simulink model "circuitbreaker_2"  (Simulink 5.1)
settings: Solver=ode23t  StartTime=0.0  StopTime=50  MaxStep=.02  RelTol=1e-3
undefined symbols (not defined in the file or in its folder): A, gcbh, powericon, sigbuilder_block
libraries: powerlib x4, simulink_extras x1, powerlib_models x1
settings Model: LastModifiedBy=Owner  BooleanDataType=on  ProdHWDeviceType=Microprocessor

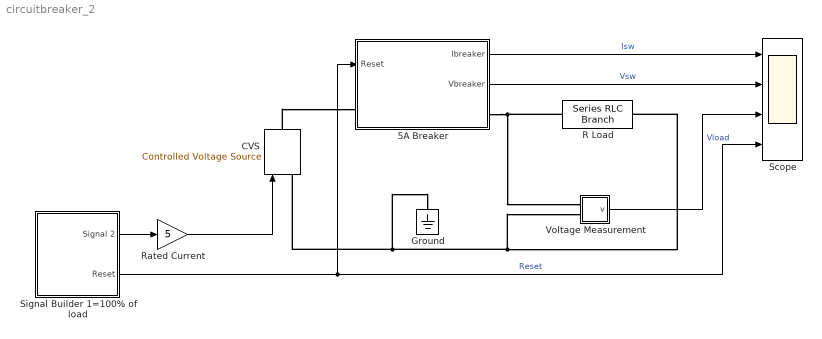
== system circuitbreaker_2 ==
  5A Breaker : Subsystem  mask{Iset=5, Tau=7}
      mask prompts: Iset "Current Rating (Amps)"; Tau "Mechanical Time Constant (Sec)"
  CVS : powerlib/Electrical Sources/Controlled Voltage Source  Description=source block  Orientation=up  Initialize=off  Amplitude=0  Phase=0  Frequency=60  Measurements=None
      settings: AttributesFormatString=\n
  Ground : powerlib/Elements/Ground  Orientation=down  PhysicalDomain=powersysdomain  SubClassName=unknown  PortType=p1  LConnTagsString=a
  R Load : powerlib/Elements/Series RLC Branch  PhysicalDomain=powersysdomain  SubClassName=unknown  PortType=p1  LConnTagsString=__new0  RConnTagsString=__new0  Resistance=1  Inductance=0  Capacitance=inf  Measurements=None
  Rated Current : Gain  Gain=5  SaturateOnIntegerOverflow=on
  Scope : Scope  NumInputPorts=4
      settings: TimeRange=50  YMin=3~-1~3~0  YMax=6~2~6~1
  Signal Builder 1=100% of load : Subsystem  Tag=STV Subsys  LoadFcn=sigbuilder_block('open',[44.25 356.25 526.5 286.5 ]);  StartFcn=sigbuilder_block('start');  StopFcn=sigbuilder_block('stop');  ClipboardFcn=sigbuilder_block('clipboard');  mask(Sigbuilder block){}
      mask help: Sigbuilder GUI
      mask init:
      | if ~strcmp(get_param(bdroot,'SimulationStatus'),'stopped') tuvar = sigbuilder_block('maskInit'); end
      settings: CopyFcn=sigbuilder_block('copy');  DeleteFcn=sigbuilder_block('delete');  ModelCloseFcn=sigbuilder_block('modelClose');  PreSaveFcn=sigbuilder_block('preSave');  NameChangeFcn=sigbuilder_block('namechange');  OpenFcn=sigbuilder_block('open',[44.25 356.25 526.5 286.5 ]);  CloseFcn=sigbuilder_block('close');
      mask Display: plot(0,0,100,100,[10,10,40,40,10],[80,20,20,80,80],[40,10],[50,50], [40,27,10],[65,72,56],[40,25,25,10],[28,28,43,43]);
  Voltage Measurement : Subsystem  Tag=PoWeRsYsTeMmEaSuReMeNt  AncestorBlock=powerlib/Measurements/Voltage Measurement  LoadFcn=powericon('psbloadfunction',gcbh,'Measurement Block','');  InitFcn=powericon('psbloadfunction',gcbh,'InitFcnOfSPSBlocks','Measurement Block');  mask(Voltage Measurement){PhasorSimulation=off, OutputType=Magnitude, PSBequivalent=1}
      mask prompts: PhasorSimulation "Phasor simulation"; OutputType "Output signal :"; PSBequivalent "Equivalent circuit"
      mask help: Ideal voltage measurement.
      mask init:
      | switch OutputType
      | case 1
      |     OutputSelection = 1;
      |     NormalMode = 2;
      |     PhasorMode = 1;
      | case 2
      |     OutputSelection =[2,3];
      |     NormalMode = 3;
      |     PhasorMode = [1,2];
      | case 3
      |     OutputSelection =[4,5];
      |     NormalMode = 3;
      |     PhasorMode = [1,2];
      | case 4
      |     OutputSelection =[4];
      |     NormalMode = 2;
      |     PhasorMode = 1;
      | end
      | %
      | if PhasorSimulation
      |     SelectionMode = PhasorMode;
      | else
      |     SelectionMode = NormalMode;
      | end
      settings: AttributesFormatString=\n  CopyFcn=powericon('psbloadfunction',gcbh,'Measurement Block','VerifyPhasor');  PreSaveFcn=powericon('psbloadfunction',gcbh,'ModelCloseFcn','');  CloseFcn=powericon('psbloadfunction',gcbh,'CloseFcn','');
      mask Help: web(psbhelp);
      mask StyleString: checkbox,popup(Complex|Real-Imag|Magnitude-Angle|Magnitude),edit
  wires:
  Voltage Measurement/1(v) -> Scope/3  "Vload"
  5A Breaker/1(Ibreaker) -> Scope/1  "Isw"
  5A Breaker/2(Vbreaker) -> Scope/2  "Vsw"
  Signal Builder 1=100% of load/1(Signal 2) -> Rated Current/1
  Rated Current/1 -> CVS/1
  Signal Builder 1=100% of load/2(Reset) -> 5A Breaker/1(Reset), Scope/4  "Reset"
  connections:
  Voltage Measurement/LConn2 -- R Load/RConn1 -- CVS/LConn1 -- Ground/LConn1
  CVS/RConn1 -- 5A Breaker/LConn1
  R Load/LConn1 -- 5A Breaker/RConn1 -- Voltage Measurement/LConn1

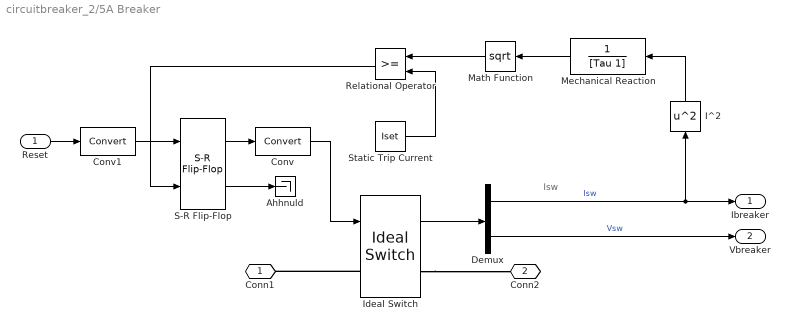
== system circuitbreaker_2/5A Breaker ==
  note: Isw
  Reset : Inport
  Ahhnuld : Terminator
  Conv : DataTypeConversion  DataType=double  SaturateOnIntegerOverflow=on
  Conv1 : DataTypeConversion  DataType=boolean  SaturateOnIntegerOverflow=on
  Demux : Demux  Outputs=2
  I^2 : Math  Orientation=up  Operator=square
  Ideal Switch : powerlib/Power Electronics/Ideal Switch  Ron=0.0001  Lon=0  IC=1  Rs=0  Cs=0  Measurements=on
      settings: AttributesFormatString=\n
  Math Function : Math  Orientation=left  Operator=sqrt
  Mechanical Reaction : TransferFcn  Orientation=left  Denominator=[Tau 1]
  Relational Operator : RelationalOperator  Orientation=left
  S-R Flip-Flop : simulink_extras/Flip Flops/S-R Flip-Flop  initial_condition=1
  "Static Trip Current " : Constant  Value=Iset
  Conn1 : PMIOPort  Port=1  Side=left
  Conn2 : PMIOPort  Orientation=left  Port=2  Side=right
  Ibreaker : Outport
  Vbreaker : Outport  Port=2
  wires:
  Ideal Switch/1 -> Demux/1
  Demux/1 -> Ibreaker/1, I^2/1  "Isw"
  Mechanical Reaction/1 -> Math Function/1
  "Static Trip Current "/1 -> Relational Operator/2
  S-R Flip-Flop/1 -> Conv/1
  Conv/1 -> Ideal Switch/1
  Demux/2 -> Vbreaker/1  "Vsw"
  Reset/1 -> Conv1/1
  Conv1/1 -> S-R Flip-Flop/1
  S-R Flip-Flop/2 -> Ahhnuld/1
  Relational Operator/1 -> S-R Flip-Flop/2
  I^2/1 -> Mechanical Reaction/1
  Math Function/1 -> Relational Operator/1
  connections:
  Ideal Switch/LConn1 -- Conn1/RConn1
  Ideal Switch/RConn1 -- Conn2/RConn1

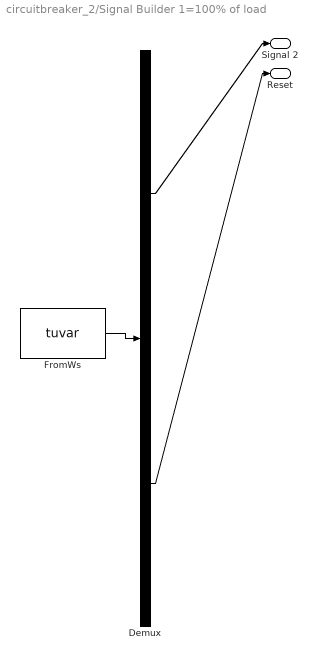
== system circuitbreaker_2/Signal Builder 1=100% of load ==
  Demux : Demux  Tag=STV Demux  Outputs=2
  FromWs : FromWorkspace  Tag=STV FromWs  VariableName=tuvar  SampleTime=0  SigBuilderData=DataTag0
      SigBuilderData=|
      | channels(1).label = 'Signal 2'
      | channels(1).allXData = {[0 10]}
      | channels(1).allYData = {[10 10]}
      | channels(2).label = 'Reset'
      | channels(2).allXData = {[0 8.92 8.92 8.98 8.98 10]}
      | channels(2).allYData = {[0 0 1 1 0 0]}
      | dataSet.timeRange = [0 10]
      | dataSet.name = 'Group 1'
  Signal 2 : Outport  Tag=STV Outport
  Reset : Outport  Tag=STV Outport  Port=2
  wires:
  FromWs/1 -> Demux/1
  Demux/1 -> Signal 2/1
  Demux/2 -> Reset/1

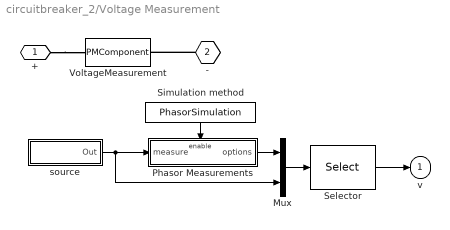
== system circuitbreaker_2/Voltage Measurement ==
  Mux : Mux  Inputs=2
  Phasor Measurements : Subsystem  TreatAsAtomicUnit=on
  Selector : Selector  Elements=SelectionMode  InputPortWidth=length(OutputSelection)+1
  Simulation method : Constant  Orientation=down  Value=PhasorSimulation
  VoltageMeasurement : PMComponent  PhysicalDomain=powersysdomain  PortType=p1  LConnTagsString=+  RConnTagsString=-
      mask Type: InnerPowersysBlock
  source : Subsystem
      mask init:
      | pss=powericon('loadsavedata','circuitbreaker_2','load');if isempty(pss),A=0;B=0;C=0;D=0;x0=0;Rswitch=0;TypeSwitch=0;Ts=0;YSwitchCurrent=-1;else,A=pss.A;B=pss.B;C=pss.C;D=pss.D;x0=pss.x0;Rswitch=pss.Rswitch;TypeSwitch=pss.TypeSwitch;Ts=0;YSwitchCurrent=pss.YSwitchCurrent;end
  + : PMIOPort  Port=1  Side=left
  - : PMIOPort  Orientation=left  Port=2  Side=left
  v : Outport  InitialOutput=0
  wires:
  Simulation method/1 -> Phasor Measurements/Enable
  Mux/1 -> Selector/1
  Phasor Measurements/1(options) -> Mux/1
  Selector/1 -> v/1
  source/1(Out) -> Phasor Measurements/1(measure), Mux/2
  connections:
  -/RConn1 -- VoltageMeasurement/RConn1
  +/RConn1 -- VoltageMeasurement/LConn1

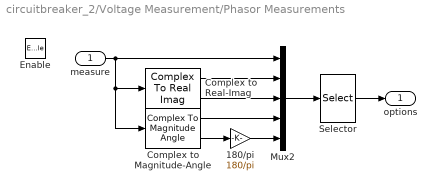
== system circuitbreaker_2/Voltage Measurement/Phasor Measurements ==
  measure : Inport
  Enable : EnablePort
  180/pi : Gain  Gain=180/pi  SaturateOnIntegerOverflow=on
  Complex to Magnitude-Angle : ComplexToMagnitudeAngle
  Complex to Real-Imag : ComplexToRealImag
  Mux2 : Mux  Inputs=5
  Selector : Selector  Elements=OutputSelection  InputPortWidth=5
  options : Outport  InitialOutput=0
  wires:
  Mux2/1 -> Selector/1
  measure/1 -> Complex to Magnitude-Angle/1, Complex to Real-Imag/1, Mux2/1
  Complex to Real-Imag/1 -> Mux2/2
  Complex to Real-Imag/2 -> Mux2/3
  Complex to Magnitude-Angle/1 -> Mux2/4
  Complex to Magnitude-Angle/2 -> 180/pi/1
  180/pi/1 -> Mux2/5
  Selector/1 -> options/1

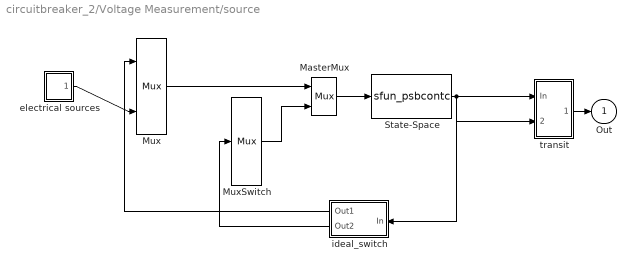
== system circuitbreaker_2/Voltage Measurement/source ==
  MasterMux : Mux  Inputs=[-1 1]
  Mux : Mux  Inputs=[1 1]
  MuxSwitch : Mux  Inputs=1
  State-Space : S-Function  FunctionName=sfun_psbcontc  Parameters=A,B,C,D,x0,Rswitch,YSwitchCurrent
  electrical sources : Subsystem
  ideal_switch : Subsystem  Orientation=left
  transit : Subsystem
  Out : Outport  InitialOutput=0
  wires:
  transit/1(Out) -> Out/1
  State-Space/1 -> transit/1(In), ideal_switch/1(In), transit/2(signals)
  MasterMux/1 -> State-Space/1
  MuxSwitch/1 -> MasterMux/2
  Mux/1 -> MasterMux/1
  ideal_switch/1(Out1) -> Mux/1
  ideal_switch/2(Out2) -> MuxSwitch/1
  electrical sources/1(Out) -> Mux/2

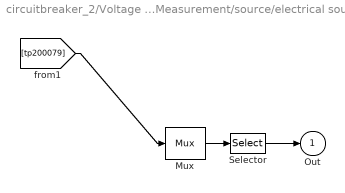
== system circuitbreaker_2/Voltage Measurement/source/electrical sources ==
  Mux : Mux  Inputs=[-1]
  Selector : Selector  InputPortWidth=2
  Out : Outport  InitialOutput=0
  wires:
  Selector/1 -> Out/1
  Mux/1 -> Selector/1
  [tp200079] -> Mux/1

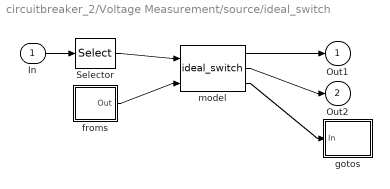
== system circuitbreaker_2/Voltage Measurement/source/ideal_switch ==
  In : Inport
  Selector : Selector  InputPortWidth=2
  froms : Subsystem
  gotos : Subsystem
  model : powerlib_models/Continuous/ideal_switch  Nsw=1  Rsw=0.0001
  Out1 : Outport  InitialOutput=0
  Out2 : Outport  Port=2  InitialOutput=0
  wires:
  In/1 -> Selector/1
  Selector/1 -> model/1
  model/1 -> Out1/1
  model/2 -> Out2/1
  model/3 -> gotos/1(In)
  froms/1(Out) -> model/2

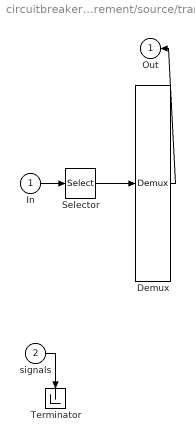
== system circuitbreaker_2/Voltage Measurement/source/transit ==
  In : Inport
  signals : Inport  Port=2
  Demux : Demux  Outputs=1
  Selector : Selector  Elements=2  InputPortWidth=2
  Terminator : Terminator
      settings: Orientation=down
  Out : Outport  Orientation=left  InitialOutput=0
  wires:
  In/1 -> Selector/1
  Selector/1 -> Demux/1
  signals/1 -> Terminator/1
  Demux/1 -> Out/1

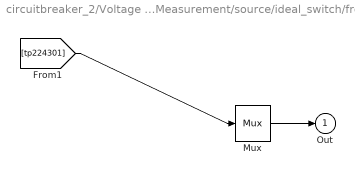
== system circuitbreaker_2/Voltage Measurement/source/ideal_switch/froms ==
  Mux : Mux  Inputs=1
  Out : Outport  InitialOutput=0
  wires:
  Mux/1 -> Out/1
  [tp224301] -> Mux/1

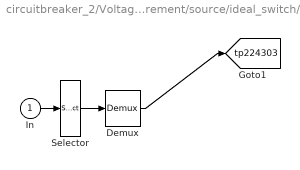
== system circuitbreaker_2/Voltage Measurement/source/ideal_switch/gotos ==
  In : Inport
  Demux : Demux  Outputs=1
  Selector : Selector  Elements=[1 2]  InputPortWidth=2
  tag scope: tp224303=global
  wires:
  In/1 -> Selector/1
  Selector/1 -> Demux/1
  Demux/1 -> [tp224303]
